simulink model "Motor_Speed_Control"  (R2021b)
settings: Solver=ode45  StartTime=0.0  StopTime=5  RelTol=1e-3
values from neighbouring files (symbols this model uses):
  b = 0.1    [Mot_spd_cntrl.mat]
  J = 0.01    [Mot_spd_cntrl.mat]
  Ke = 0.01    [Mot_spd_cntrl.mat]
  Kt = 0.01    [Mot_spd_cntrl.mat]
  L = 0.5    [Mot_spd_cntrl.mat]
  R = 1    [Mot_spd_cntrl.mat]
  V = 27    [Mot_spd_cntrl.mat]
settings Model: Creator=Manmath Kharade  LastModifiedBy=Manmath Kharade
settings OptimizationCC: DefaultParameterBehavior=Inlined  UseDivisionForNetSlopeComputation=on  EnhancedBackFolding=on  PassReuseOutputArgsAs=Individual arguments  ZeroExternalMemoryAtStartup=off  ZeroInternalMemoryAtStartup=off  OptimizeBlockOrder=speed  DifferentSizesBufferReuse=on  OptimizationCustomize=off  EfficientTunableParamExpr=on
settings DebuggingCC: AlgebraicLoopMsg=none  ParameterTunabilityLossMsg=error
settings HardwareCC: TargetBitPerPointer=64  TargetBitPerSizeT=64  TargetBitPerPtrDiffT=64  TargetLongLongMode=on  TargetIntDivRoundTo=Zero  TargetEndianess=LittleEndian  TargetWordSize=64  TargetHWDeviceType=MATLAB Host  ProdEqTarget=off
settings ModelReferenceCC: ModelReferenceMinAlgLoopOccurrences=on
settings SFSimCC: MATLABDynamicMemAlloc=off
settings RTWCC: Description=Embedded Coder  SystemTargetFile=ert.tlc  GenCodeOnly=on  PackageGeneratedCodeAndArtifacts=on  PackageName=Mtr_spd_cntrl_code  TemplateMakefile=ert_default_tmf  GenerateReport=on  LaunchReport=on  CheckMdlBeforeBuild=Warning
settings CodeAppCC: ForceParamTrailComments=on  IgnoreCustomStorageClasses=off  OperatorAnnotations=on  SimulinkDataObjDesc=on  SFDataObjDesc=on  InsertBlockDesc=on
settings ERTTargetCC: TargetLangStandard=C99 (ISO)  GenerateSampleERTMain=on  InlinedParameterPlacement=NonHierarchical  ERTCustomFileTemplate=example_file_process.tlc

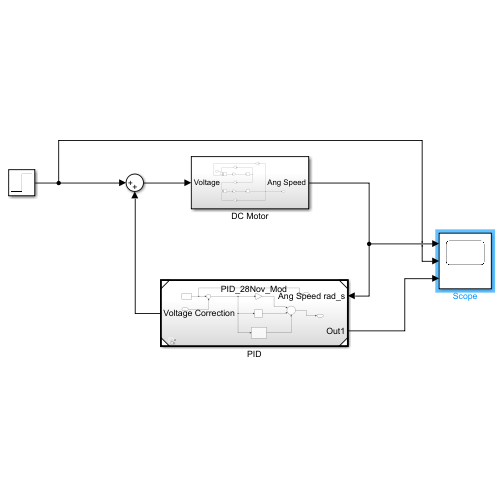
[thumbnail: Simulink's stored preview of the top-level diagram]
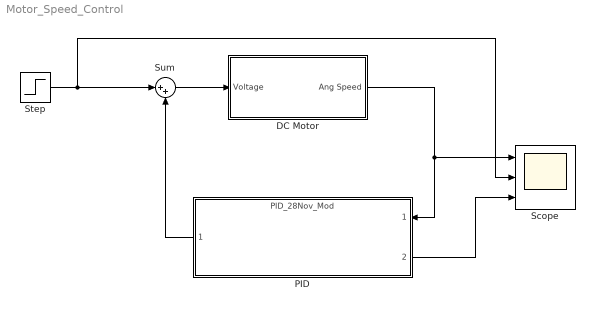
== system Motor_Speed_Control ==
  DC Motor : Subsystem
  PID : ModelReference  ModelNameDialog=PID_28Nov_Mod.slx  SimulationMode=Normal  ModelReferenceVersion=1.11
      settings: PortSchema="{\"entries\":[{\"content\":{\"sides\":[{\"content\":{\"connectorIds\":[\"In1\",\"Out2\"]},\"type\":\"ConnectorPlacement.EquallySpacedRectSide\",\"uuid\":\"ad25bb13-e720-4a00-b2f1-361fba6a337d\"},{\"content\":{\"connectorIds\":[\"Out1\"],\"side\":\"RIGHT\"},\"type\":\"ConnectorPlacement.EquallySpacedRectSide\",\"uuid\":\"640f5347-1387-4770-be32-b13457e3f63e\"},{\"content\":{\"connectorIds\":[],\"side\":\"TOP\"},\"type\":\"ConnectorPlacement.EquallySpacedRectSide\",\"uuid\":\"4c14a7dd-82ea-4f02-9096-9ce4fd6786ed\"}]},\"type\":\"ConnectorPlacement.EquallySpacedConnector\",\"uuid\":\"977545e8-18f2-4508-aeda-43b8e12f48a2\"}],\"packageUris\":[\"http://schema.mathworks.com/mf0/Connector/R2020b\"],\"version\":\"1.0\"}"
  Scope : Scope  NumInputPorts=3
  Step : Step  Time=0  After=V  SampleTime=0
  Sum : Sum  Inputs=|++
  wires:
  Step/1 -> Scope/2, Sum/1
  DC Motor/1(Ang Speed) -> PID/1, Scope/1
  Sum/1 -> DC Motor/1(Voltage)
  PID/1 -> Sum/2
  PID/2 -> Scope/3

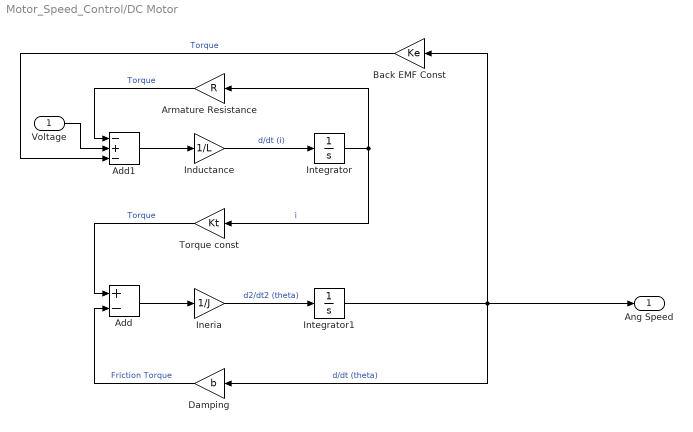
== system Motor_Speed_Control/DC Motor ==
  Voltage : Inport
  Add : Sum  Inputs=+-
  Add1 : Sum  Inputs=-+-
  Armature Resistance : Gain  Gain=R
  Back EMF Const : Gain  Gain=Ke
  Damping : Gain  Gain=b
  Inductance : Gain  Gain=1/L
  Ineria : Gain  Gain=1/J
  Integrator : Integrator
  Integrator1 : Integrator
  Torque const : Gain  Gain=Kt
  Ang Speed : Outport
  wires:
  Damping/1 -> Add/2  "Friction Torque"
  Add1/1 -> Inductance/1
  Integrator1/1 -> Damping/1, Ang Speed/1, Back EMF Const/1  "d/dt (theta)"
  Torque const/1 -> Add/1  "Torque"
  Armature Resistance/1 -> Add1/1  "Torque"
  Ineria/1 -> Integrator1/1  "d2/dt2 (theta)"
  Voltage/1 -> Add1/2
  Integrator/1 -> Torque const/1, Armature Resistance/1  "i"
  Inductance/1 -> Integrator/1  "d/dt (i)"
  Add/1 -> Ineria/1
  Back EMF Const/1 -> Add1/3  "Torque"
